simulink model "sl_ps_converter_u1"  (R2024b)
settings: Solver=VariableStepAuto  StartTime=0.0  StopTime=10.0  RelTol=1e-3
libraries: fl_lib x2, nesl_utility x1
settings Model: Creator=uditpant  LastModifiedBy=uditpant

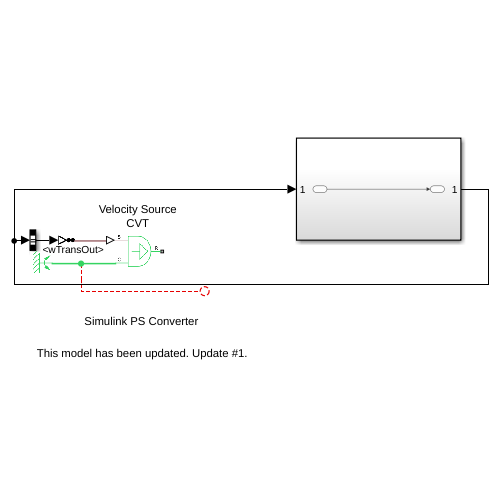
[thumbnail: Simulink's stored preview of the top-level diagram]
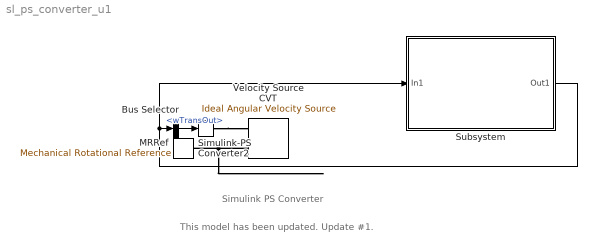
== system sl_ps_converter_u1 ==
  note: This model has been updated. Update #1.
  note: Simulink PS Converter
  Bus Selector : BusSelector  OutputSignals=Operator.wTransOut
  MRRef : fl_lib/Mechanical/Rotational Elements/Mechanical Rotational Reference
  Simulink-PS Converter2 : nesl_utility/Simulink-PS Converter  PhysicalDomain=network_engine_domain  SubClassName=ps_input  LeftPortType=input  RightPortType=output  PseudoPeriodic=off  Frequencies=[]  NoiseDistribution=none  NoiseParameters=[]  Unit=rpm  AffineConversion=off  FilteringAndDerivatives=filter  SimscapeFilterOrder=2  InputFilterTimeConstant=0.1  UdotUserProvided=0
  Subsystem : Subsystem
  Velocity Source CVT : fl_lib/Mechanical/Mechanical Sources/Ideal Angular Velocity Source
  wires:
  Bus Selector/1 -> Simulink-PS Converter2/1  "<wTransOut>"
  Subsystem/1(Out1) -> Subsystem/1(In1), Bus Selector/1
  connections:
  Velocity Source CVT/RConn2 -- MRRef/LConn1
  Simulink-PS Converter2/RConn1 -- Velocity Source CVT/RConn1

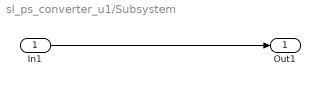
== system sl_ps_converter_u1/Subsystem ==
  In1 : Inport
  Out1 : Outport
  wires:
  In1/1 -> Out1/1
